simulink model "Lab2_Task_5678"  (R2023b)
settings: Solver=VariableStepAuto  StartTime=0.0  StopTime=10.0  RelTol=1e-3
undefined symbols (not defined in the file or in its folder): angdiff, Angular, Linear
libraries: robotlib x4, robotcorelib x1, simulink_extras x1, simulink x1
settings Model: Creator=Sina  LastModifiedBy=hampu
settings SolverCC: AlgebraicLoopSolver=TrustRegion
settings DataIOCC: ReturnWorkspaceOutputs=off
settings DebuggingCC: UnconnectedInputMsg=warning  UnconnectedOutputMsg=warning  UnconnectedLineMsg=warning  ArithmeticOperatorsInVariantConditions=warning
settings ModelReferenceCC: EnableRefExpFcnMdlSchedulingChecks=on
settings SFSimCC: SimUseLocalCustomCode=off  CustomCodeUndefinedFunction=UseInterfaceOnly
settings RTWCC: RTWUseLocalCustomCode=off

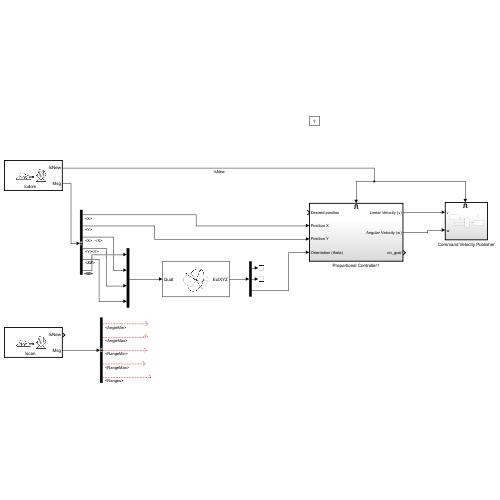
[thumbnail: Simulink's stored preview of the top-level diagram]
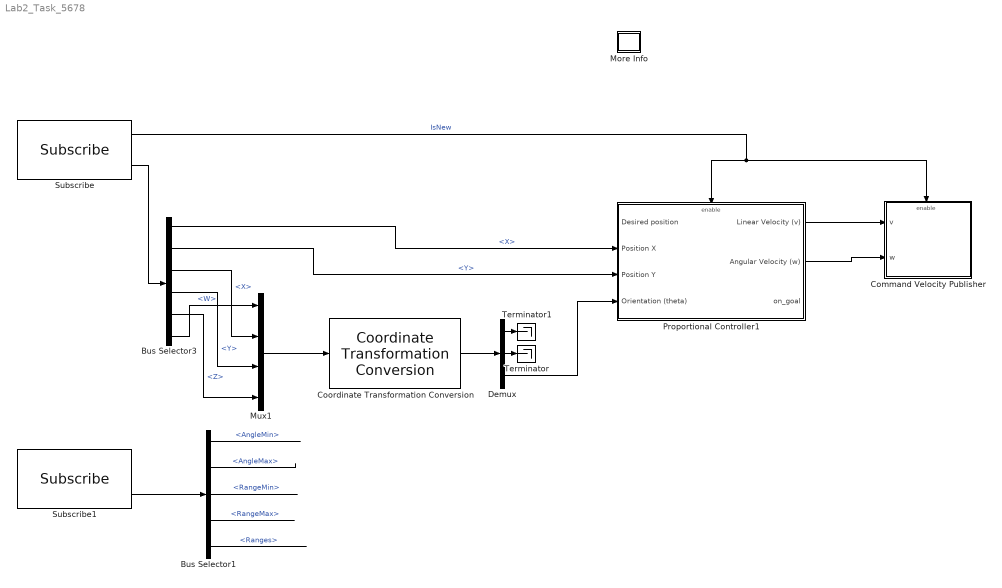
== system Lab2_Task_5678 ==
  Bus Selector1 : BusSelector  OutputSignals=AngleMin,AngleMax,RangeMin,RangeMax,Ranges
  Bus Selector3 : BusSelector  OutputSignals=Pose.Pose.Position.X,Pose.Pose.Position.Y,Pose.Pose.Orientation.X,Pose.Pose.Orientation.Y,Pose.Pose.Orientation.Z,Pose.Pose.Orientation.W
  Command Velocity Publisher : Subsystem
  Coordinate Transformation Conversion : robotcorelib/Coordinate Transformation Conversion  InputRepresentation=Quaternion  InputEulerSequence=ZYX  ShowTrVecInputPort=on  OutputRepresentation=Euler Angles  OutputEulerSequence=XYZ  ShowTrVecOutputPort=on  SimulateUsing=Interpreted execution
      settings: LibrarySourceBlock=roslib/Utilities/Coordinate Transformation Conversion
  Demux : Demux  Outputs=3
  More Info : Subsystem
      settings: OpenFcn=showdemo(bdroot(gcb))
      mask Display: disp('?')
  Mux1 : Mux
  Proportional Controller1 : Subsystem
  Subscribe : robotlib/Subscribe  topicSource=Select from ROS network  topic=/odom  messageType=nav_msgs/Odometry  SampleTime=-1  legacyBusStruct=off  messageQueueLength=51
  Subscribe1 : robotlib/Subscribe  topicSource=Select from ROS network  topic=/scan  messageType=sensor_msgs/LaserScan  SampleTime=-1  legacyBusStruct=off  messageQueueLength=51
  Terminator : Terminator
  Terminator1 : Terminator
  wires:
  Bus Selector3/2 -> Proportional Controller1/3(Position Y)  "<Y>"
  Bus Selector3/1 -> Proportional Controller1/2(Position X)  "<X>"
  Proportional Controller1/2(Angular Velocity (w)) -> Command Velocity Publisher/2(w)
  Subscribe/1 -> Proportional Controller1/Enable, Command Velocity Publisher/Enable  "IsNew"
  Proportional Controller1/1(Linear Velocity (v)) -> Command Velocity Publisher/1(v)
  Subscribe/2 -> Bus Selector3/1
  Bus Selector1/3 -> ?  "<RangeMin>"
  Bus Selector1/4 -> ?  "<RangeMax>"
  Bus Selector1/2 -> ?  "<AngleMax>"
  Bus Selector1/5 -> ?  "<Ranges>"
  Subscribe1/2 -> Bus Selector1/1
  Bus Selector1/1 -> ?  "<AngleMin>"
  Demux/2 -> Terminator/1
  Bus Selector3/4 -> Mux1/3  "<Y>"
  Coordinate Transformation Conversion/1 -> Demux/1
  Bus Selector3/6 -> Mux1/1  "<W>"
  Mux1/1 -> Coordinate Transformation Conversion/1
  Demux/1 -> Terminator1/1
  Demux/3 -> Proportional Controller1/4(Orientation (theta))
  Bus Selector3/5 -> Mux1/4  "<Z>"
  Bus Selector3/3 -> Mux1/2  "<X>"

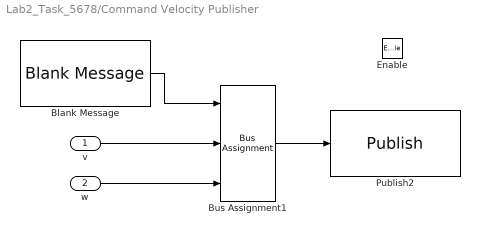
== system Lab2_Task_5678/Command Velocity Publisher ==
  v : Inport
  w : Inport  Port=2
  Enable : EnablePort
  Blank Message : robotlib/Blank Message  SourceLibraryInfo=This block requires Robotics System Toolbox  messageType=geometry_msgs/Twist  SampleTime=inf
  Bus Assignment1 : BusAssignment  DialogController=Simulink.DDGSource_BusAssignment  AssignedSignals=Linear.X,Angular.Z
  Publish2 : robotlib/Publish  SourceLibraryInfo=This block requires Robotics System Toolbox  topicSource=Select from ROS network  topic=/cmd_vel  messageType=geometry_msgs/Twist  messageQueueLength=105
  wires:
  Bus Assignment1/1 -> Publish2/1
  Blank Message/1 -> Bus Assignment1/1
  v/1 -> Bus Assignment1/2
  w/1 -> Bus Assignment1/3

== system Lab2_Task_5678/More Info ==

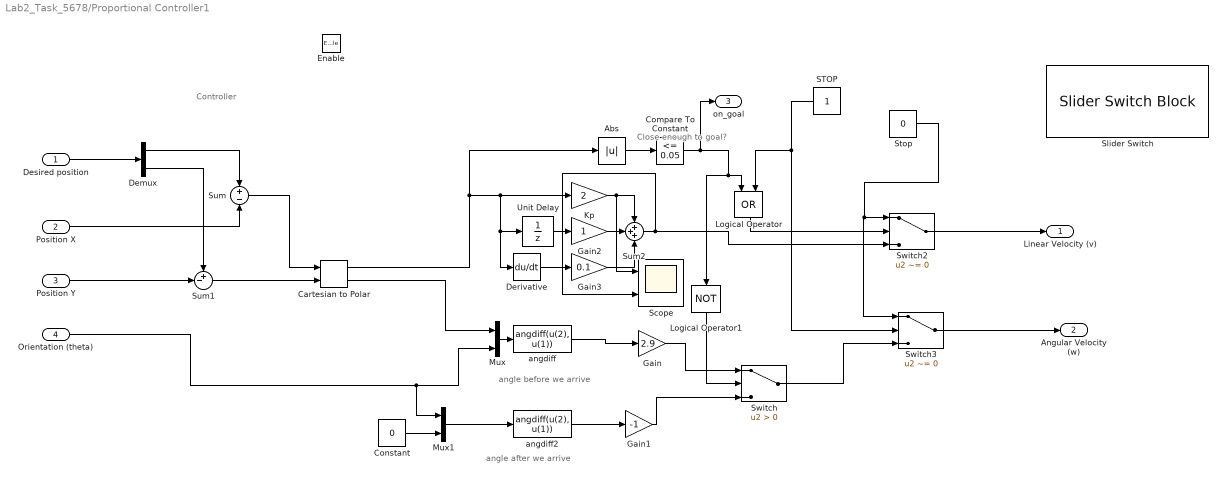
== system Lab2_Task_5678/Proportional Controller1 ==
  note: angle after we arrive
  note: Controller
  note: Close enough to goal?
  note: angle before we arrive
  Desired position : Inport
  Position X : Inport  Port=2
  Position Y : Inport  Port=3
  Orientation (theta) : Inport  Port=4
  Enable : EnablePort
  Abs : Abs  SaturateOnIntegerOverflow=off
  Cartesian to Polar : simulink_extras/Transformations/Cartesian to Polar
  Compare To Constant : simulink/Logic and Bit Operations/Compare To Constant  relop=<=  const=0.05  OutDataTypeStr=boolean
  Constant : Constant  Value=0
  Demux : Demux  Outputs=2
  Derivative : Derivative
  Gain : Gain  Gain=2.9
  Gain1 : Gain  Gain=-1
  Gain2 : Gain
  Gain3 : Gain  Gain=0.1
  Kp : Gain  Gain=2
  Logical Operator : Logic  Operator=OR  AllPortsSameDT=off  OutDataTypeStr=boolean
  Logical Operator1 : Logic  Operator=NOT  AllPortsSameDT=off  OutDataTypeStr=boolean
  Mux : Mux  Inputs=2
  Mux1 : Mux  Inputs=2
  "STOP " : Constant
  Scope : Scope  NumInputPorts=2
  Slider Switch : SliderSwitchBlock
      settings: Values={{'Off', 'On'}, [0 1]}
  Stop : Constant  Value=0
  Sum : Sum  Inputs=+-
  Sum1 : Sum  Inputs=+-|
  Sum2 : Sum  Inputs=+++
  Switch : Switch  Criteria=u2 > Threshold  SaturateOnIntegerOverflow=off  InputSameDT=off
  Switch2 : Switch  Criteria=u2 ~= 0  SaturateOnIntegerOverflow=off  InputSameDT=off
  Switch3 : Switch  Criteria=u2 ~= 0  SaturateOnIntegerOverflow=off  InputSameDT=off
  Unit Delay : UnitDelay  SampleTime=-1  HasFrameUpgradeWarning=on
  angdiff : MATLABFcn  MATLABFcn=angdiff(u(2), u(1))
  angdiff2 : MATLABFcn  MATLABFcn=angdiff(u(2), u(1))
  Linear Velocity (v) : Outport  VectorParamsAs1DForOutWhenUnconnected=off
  Angular Velocity (w) : Outport  Port=2  VectorParamsAs1DForOutWhenUnconnected=off
  on_goal : Outport  Port=3
  wires:
  Cartesian to Polar/2 -> Mux/1
  Switch2/1 -> Linear Velocity (v)/1
  Logical Operator/1 -> Switch2/2
  Gain1/1 -> Switch/3
  Demux/2 -> Sum1/1
  Kp/1 -> Sum2/1, Scope/1
  Desired position/1 -> Demux/1
  Mux1/1 -> angdiff2/1
  angdiff2/1 -> Gain1/1
  Sum/1 -> Cartesian to Polar/1
  Mux/1 -> angdiff/1
  Switch3/1 -> Angular Velocity (w)/1
  Position X/1 -> Sum/2
  Abs/1 -> Compare To Constant/1
  Position Y/1 -> Sum1/2
  Sum1/1 -> Cartesian to Polar/2
  Gain/1 -> Switch/1
  angdiff/1 -> Gain/1
  Switch/1 -> Switch3/3
  Stop/1 -> Switch3/1, Switch2/1
  Orientation (theta)/1 -> Mux1/1, Mux/2
  Logical Operator1/1 -> Switch/2
  Demux/1 -> Sum/1
  Compare To Constant/1 -> on_goal/1, Logical Operator1/1, Logical Operator/1
  "STOP "/1 -> Switch3/2, Logical Operator/2
  Constant/1 -> Mux1/2
  Unit Delay/1 -> Gain2/1
  Derivative/1 -> Gain3/1
  Cartesian to Polar/1 -> Abs/1, Unit Delay/1, Derivative/1, Kp/1
  Gain2/1 -> Sum2/2
  Gain3/1 -> Sum2/3
  Sum2/1 -> Scope/2, Switch2/3
